simulink model "Cruise_Control"  (R2022b)
settings: configuration reference "CommonModelConfiguration" (kept outside this file)
undefined symbols (not defined in the file): cc_param_23, LCFG_ActivationDeactivation, LCFG_CC_IntStsDelay, LCFG_CC_Tmr1, LCFG_CC_Tmr2, LCFG_DSF_Timeout
settings Model: Creator=RPETE142  LastModifiedBy=OTHOMSO1
settings ConfigSetRef: SourceName=CommonModelConfiguration  SourceLocation=Base Workspace

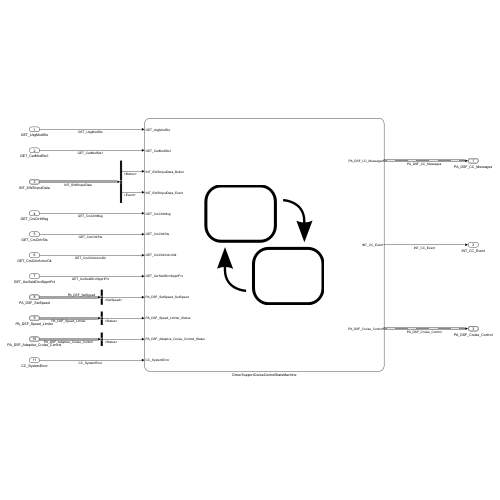
[thumbnail: Simulink's stored preview of the top-level diagram]
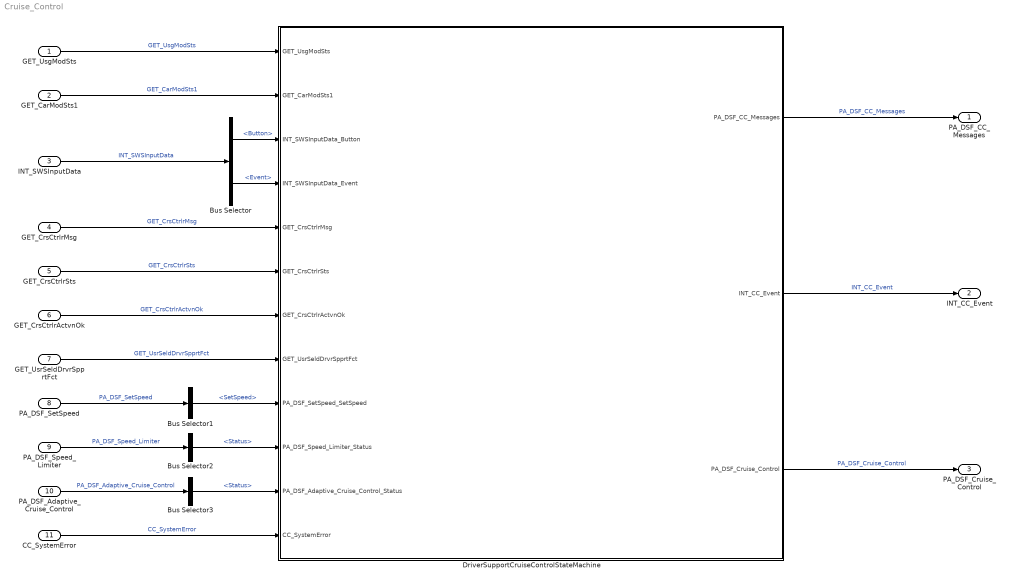
== system Cruise_Control ==
  GET_UsgModSts : Inport  OutDataTypeStr=Enum: UsgModSts1
  GET_CarModSts1 : Inport  Port=2  OutDataTypeStr=Enum: CarModSts1
  INT_SWSInputData : Inport  Port=3  OutDataTypeStr=Bus: SWSInputData  LockScale=on
  GET_CrsCtrlrMsg : Inport  Port=4  OutDataTypeStr=Enum: CrsCtrlrMsg1
  GET_CrsCtrlrSts : Inport  Port=5  OutDataTypeStr=Enum: CrsCtrlrSts1
  GET_CrsCtrlrActvnOk : Inport  Port=6  OutDataTypeStr=Enum: OnOff1
  GET_UsrSeldDrvrSpprtFct : Inport  Port=7  OutDataTypeStr=Enum: DrvrSpprtFct
  PA_DSF_SetSpeed : Inport  Port=8  OutDataTypeStr=Bus: PA_StatusAndValueAndDoubleAndDouble
  PA_DSF_Speed_Limiter : Inport  Port=9  OutDataTypeStr=Bus: PA_DSF
  PA_DSF_Adaptive_Cruise_Control : Inport  Port=10  OutDataTypeStr=Bus: PA_DSF_ACC
  CC_SystemError : Inport  Port=11  OutDataTypeStr=boolean
  Bus Selector : BusSelector  OutputSignals=Button,Event
  Bus Selector1 : BusSelector  OutputSignals=SetSpeed
  Bus Selector2 : BusSelector  OutputSignals=Status
  Bus Selector3 : BusSelector  OutputSignals=Status
  "DriverSupportCruiseControlStateMachine " : Stateflow chart  TreatAsAtomicUnit=on
  PA_DSF_CC_Messages : Outport  OutDataTypeStr=Bus: PA_DSF_Message  VectorParamsAs1DForOutWhenUnconnected=off  LockScale=on
  INT_CC_Event : Outport  Port=2  OutDataTypeStr=Enum: E_DSF_Event  VectorParamsAs1DForOutWhenUnconnected=off
  PA_DSF_Cruise_Control : Outport  Port=3  OutDataTypeStr=Bus: PA_DSF  VectorParamsAs1DForOutWhenUnconnected=off
  wires:
  GET_UsgModSts/1 -> "DriverSupportCruiseControlStateMachine "/1(GET_UsgModSts)  "GET_UsgModSts"
  GET_CarModSts1/1 -> "DriverSupportCruiseControlStateMachine "/2(GET_CarModSts1)  "GET_CarModSts1"
  GET_CrsCtrlrMsg/1 -> "DriverSupportCruiseControlStateMachine "/5(GET_CrsCtrlrMsg)  "GET_CrsCtrlrMsg"
  GET_CrsCtrlrActvnOk/1 -> "DriverSupportCruiseControlStateMachine "/7(GET_CrsCtrlrActvnOk)  "GET_CrsCtrlrActvnOk"
  GET_CrsCtrlrSts/1 -> "DriverSupportCruiseControlStateMachine "/6(GET_CrsCtrlrSts)  "GET_CrsCtrlrSts"
  "DriverSupportCruiseControlStateMachine "/1(PA_DSF_CC_Messages) -> PA_DSF_CC_Messages/1  "PA_DSF_CC_Messages"
  "DriverSupportCruiseControlStateMachine "/2(INT_CC_Event) -> INT_CC_Event/1  "INT_CC_Event"
  "DriverSupportCruiseControlStateMachine "/3(PA_DSF_Cruise_Control) -> PA_DSF_Cruise_Control/1  "PA_DSF_Cruise_Control"
  GET_UsrSeldDrvrSpprtFct/1 -> "DriverSupportCruiseControlStateMachine "/8(GET_UsrSeldDrvrSpprtFct)  "GET_UsrSeldDrvrSpprtFct"
  PA_DSF_SetSpeed/1 -> Bus Selector1/1  "PA_DSF_SetSpeed"
  PA_DSF_Speed_Limiter/1 -> Bus Selector2/1  "PA_DSF_Speed_Limiter"
  PA_DSF_Adaptive_Cruise_Control/1 -> Bus Selector3/1  "PA_DSF_Adaptive_Cruise_Control"
  CC_SystemError/1 -> "DriverSupportCruiseControlStateMachine "/12(CC_SystemError)  "CC_SystemError"
  INT_SWSInputData/1 -> Bus Selector/1  "INT_SWSInputData"
  Bus Selector/2 -> "DriverSupportCruiseControlStateMachine "/4(INT_SWSInputData_Event)  "<Event>"
  Bus Selector/1 -> "DriverSupportCruiseControlStateMachine "/3(INT_SWSInputData_Button)  "<Button>"
  Bus Selector1/1 -> "DriverSupportCruiseControlStateMachine "/9(PA_DSF_SetSpeed_SetSpeed)  "<SetSpeed>"
  Bus Selector2/1 -> "DriverSupportCruiseControlStateMachine "/10(PA_DSF_Speed_Limiter_Status)  "<Status>"
  Bus Selector3/1 -> "DriverSupportCruiseControlStateMachine "/11(PA_DSF_Adaptive_Cruise_Control_Status)  "<Status>"

== stateflow chart Cruise_Control/DriverSupportCruiseControlStateMachine  ==
  state CARCONFIG_INVALID
    entry:
    INT_CC_Event = E_DSF_Event.NoReq;
    PA_DSF_Cruise_Control.Status=E_CommonStatus.NotPresent;
    PA_DSF_Cruise_Control.Value=E_DSF_Value.DSF_Selected;
    PA_DSF_CC_Messages.Status = E_CommonStatus.NotPresent;
    PA_DSF_CC_Messages.Value = E_DSF_Messages.Messages_Off;
  state SYSTEM_OK
    state isActive = activationCheck [function]
      (default) -> (junction 35)
      (junction 35) -> (junction 28) [order 1] : [GET_UsgModSts == UsgModSts1.UsgModSts1_UsgModDrvg && ...
          | (GET_CarModSts1 == CarModSts1.CarModSts1_CarModNorm ||...
          | GET_CarModSts1 == CarModSts1.CarModSts1_CarModDyno) &&...
          | (GET_UsrSeldDrvrSpprtFct==DrvrSpprtFct.DrvrSpprtFct_CC ||...
          | PA_DSF_Cruise_Control.Value==E_DSF_Value.DSF_Active) &&...
          | PA_DSF_Speed_Limiter_Status ~=E_CommonStatus.Available &&...
          | PA_DSF_Adaptive_Cruise_Control_Status~=E_CommonStatus.Available]
      (junction 35) -> (junction 29) [order 2] : {isActive = false;}
      (junction 28) -> (junction 30) : {isActive = true;}
      (junction 30) -> (junction 29)
      (junction 29) -> (junction 31)
    state NOT_ACTIVE
      entry:
      INT_CC_Event = E_DSF_Event.NoReq;
      PA_DSF_Cruise_Control.Status=E_CommonStatus.Disabled;
      PA_DSF_CC_Messages.Status = E_CommonStatus.Disabled;
      state MESSAGES_OFF
        entry:
        PA_DSF_CC_Messages.Value=E_DSF_Messages.Messages_Off;
        PA_DSF_Cruise_Control.Value=E_DSF_Value.DSF_Selected;
      state CANCEL_WARNING
        entry:
        PA_DSF_CC_Messages.Value=E_DSF_Messages.Messages_CancelWarning;
        PA_DSF_Cruise_Control.Value=E_DSF_Value.DSF_Selected;
      (default) -> (junction 1215)
      (junction 1215) -> (junction 1214) [order 1] : [PA_DSF_Cruise_Control.Value==E_DSF_Value.DSF_Active]
      (junction 1215) -> MESSAGES_OFF [order 2]
      (junction 1214) -> SYSTEM_OK.NOT_ACTIVE.CANCEL_WARNING
      SYSTEM_OK.NOT_ACTIVE.CANCEL_WARNING -> MESSAGES_OFF : [after(LCFG_DSF_Timeout, sec)]
    state PENDING
    state PENDING1
    state ACTIVE
      state MESSAGES [parallel]
        entry:
        PA_DSF_CC_Messages.Status = E_CommonStatus.Available;
        settings: executionOrder=1
        state retVal = ccMessages [function]
          state retVal2 = ccActivationReq [function]
            (default) -> (junction 1536)
            (junction 1536) -> (junction 1537) [order 1] : [(GET_CrsCtrlrSts ~= CrsCtrlrSts1.CrsCtrlrSts1_Actv)...
                | && (GET_CrsCtrlrActvnOk == OnOff1.OnOff1_Off)...
                | && (INT_SWSInputData_Button ==  E_SWSButton.BtnL1Req)...
                | && hasChangedTo(INT_SWSInputData_Event,E_SWSEvent.Push)]
            (junction 1536) -> (junction 1539) [order 2]
            (junction 1537) -> (junction 1538)
            (junction 1539) -> (junction 1538) [order 1] : [(GET_CrsCtrlrSts ~= CrsCtrlrSts1.CrsCtrlrSts1_Actv)...
                | && (GET_CrsCtrlrActvnOk == OnOff1.OnOff1_Off)...
                | && (INT_SWSInputData_Button ==  E_SWSButton.BtnL5Req)...
                | && hasChangedTo(INT_SWSInputData_Event,E_SWSEvent.Push)...
                | && (PA_DSF_SetSpeed_SetSpeed~=0)]
            (junction 1538) -> (junction 1540) : {retVal2 = true;}
            (junction 1539) -> (junction 1541) [order 2] : {retVal2 = false;}
            (junction 1540) -> (junction 1541)
            (junction 1541) -> (junction 1542)
          (default) -> (junction 1502)
          (junction 1502) -> (junction 1487) [order 1] : [hasChangedTo(GET_CrsCtrlrMsg, CrsCtrlrMsg1.CrsCtrlrMsg1_CrsCtrlrCncl)]
              | {PA_DSF_CC_Messages.Value = E_DSF_Messages.Messages_CancelWarning;}
          (junction 1502) -> (junction 1504) [order 2]
          (junction 1487) -> (junction 1484)
          (junction 1504) -> (junction 1484) [order 1] : [hasChangedTo(GET_CrsCtrlrMsg, CrsCtrlrMsg1.CrsCtrlrMsg1_CrsCtrlrCnclSpdLoLimExcdd)]
              | {PA_DSF_CC_Messages.Value = E_DSF_Messages.Messages_CancelLowSpeed;}
          (junction 1504) -> (junction 1506) [order 2]
          (junction 1484) -> (junction 1456)
          (junction 1506) -> (junction 1456) [order 1] : [hasChangedTo(GET_CrsCtrlrMsg, CrsCtrlrMsg1.CrsCtrlrMsg1_OvrdTiMaxExcdd)]
              | {PA_DSF_CC_Messages.Value = E_DSF_Messages.Messages_CancelMaxOverride;}
          (junction 1506) -> (junction 1508) [order 2]
          (junction 1456) -> (junction 1494)
          (junction 1508) -> (junction 1510) [order 1] : [ccActivationReq()]
          (junction 1510) -> (junction 1494) [order 1] : [(GET_CrsCtrlrMsg == CrsCtrlrMsg1.CrsCtrlrMsg1_CrsCtrlrInhb)]
              | {PA_DSF_CC_Messages.Value = E_DSF_Messages.Messages_Unavailable;}
          (junction 1508) -> (junction 1517) [order 2]
          (junction 1510) -> (junction 1512) [order 2]
          (junction 1494) -> (junction 1463)
          (junction 1512) -> (junction 1463) [order 1] : [(GET_CrsCtrlrMsg == CrsCtrlrMsg1.CrsCtrlrMsg1_SpdLoLimExcdd)]
              | {PA_DSF_CC_Messages.Value = E_DSF_Messages.Messages_UnavailableLowSpeed;}
          (junction 1512) -> (junction 1515) [order 2]
          (junction 1463) -> (junction 1458)
          (junction 1515) -> (junction 1517) [order 2]
          (junction 1515) -> (junction 1458) [order 1] : [(GET_CrsCtrlrMsg == CrsCtrlrMsg1.CrsCtrlrMsg1_DrvModSeldNotOk)]
              |  {PA_DSF_CC_Messages.Value = E_DSF_Messages.Messages_UnavailableDriveMode;}
          (junction 1517) -> (junction 1533) : {retVal = false;}
          (junction 1458) -> (junction 1529) : {retVal = true;}
          (junction 1529) -> (junction 1533)
          (junction 1533) -> (junction 1531)
        state HIDE_MESSAGES
          entry: PA_DSF_CC_Messages.Value = E_DSF_Messages.Messages_Off;
        state SHOW_MESSAGES
        (default) -> HIDE_MESSAGES
        HIDE_MESSAGES -> SHOW_MESSAGES : [ccMessages()]
        SHOW_MESSAGES -> HIDE_MESSAGES [order 2] : [after(LCFG_DSF_Timeout,sec) ||...
            |  (GET_CrsCtrlrMsg == CrsCtrlrMsg1.CrsCtrlrMsg1_BrkOvrheatd) || ...
            | hasChangedTo(GET_CrsCtrlrSts,CrsCtrlrSts1.CrsCtrlrSts1_Actv)]
        SHOW_MESSAGES -> SHOW_MESSAGES [order 1] : [ccMessages()]
      state CC [parallel]
        entry: PA_DSF_Cruise_Control.Status=E_CommonStatus.Available;
        settings: executionOrder=2
        state STANDBY
          entry:
          PA_DSF_Cruise_Control.Value=E_DSF_Value.DSF_Standby;
          state NO_EVENT
            entry: INT_CC_Event=E_DSF_Event.NoReq;
          state EVENT
          (default) -> SYSTEM_OK.ACTIVE.CC.STANDBY.EVENT
          SYSTEM_OK.ACTIVE.CC.STANDBY.EVENT -> SYSTEM_OK.ACTIVE.CC.STANDBY.NO_EVENT : [after(LCFG_ActivationDeactivation,sec)]
        state SELECTED
          entry:
          PA_DSF_Cruise_Control.Value=E_DSF_Value.DSF_Selected;
        state ON
          entry:
          PA_DSF_Cruise_Control.Value=E_DSF_Value.DSF_Active;
          state NO_EVENT
            entry: INT_CC_Event=E_DSF_Event.NoReq;
          state EVENT
          (default) -> SYSTEM_OK.ACTIVE.CC.ON.EVENT
          SYSTEM_OK.ACTIVE.CC.ON.EVENT -> SYSTEM_OK.ACTIVE.CC.ON.NO_EVENT : [after(LCFG_ActivationDeactivation,sec)]
        (default) -> SELECTED
        SELECTED -> ON [order 2] : [(after(LCFG_CC_IntStsDelay, sec) &&...
            | GET_CrsCtrlrSts==CrsCtrlrSts1.CrsCtrlrSts1_Actv)]
        SELECTED -> ON [order 1] : [INT_SWSInputData_Button==E_SWSButton.BtnL1Req &&...
            | hasChangedTo(INT_SWSInputData_Event,E_SWSEvent.Push) &&...
            | GET_CrsCtrlrActvnOk==OnOff1.OnOff1_On]
            | {INT_CC_Event=E_DSF_Event.Activation;}
        STANDBY -> ON [order 3] : [(after(LCFG_CC_IntStsDelay, sec) &&...
            | GET_CrsCtrlrSts==CrsCtrlrSts1.CrsCtrlrSts1_Actv)]
        STANDBY -> ON [order 1] : [INT_SWSInputData_Button==E_SWSButton.BtnL1Req &&...
            | hasChangedTo(INT_SWSInputData_Event,E_SWSEvent.Push) &&...
            | GET_CrsCtrlrActvnOk==OnOff1.OnOff1_On &&...
            | INT_CC_Event==E_DSF_Event.NoReq]
            | {INT_CC_Event=E_DSF_Event.Activation;}
        STANDBY -> ON [order 2] : [INT_SWSInputData_Button==E_SWSButton.BtnL5Req &&...
            | hasChangedTo(INT_SWSInputData_Event, E_SWSEvent.Push) &&...
            | GET_CrsCtrlrActvnOk==OnOff1.OnOff1_On &&...
            | PA_DSF_SetSpeed_SetSpeed~=0 &&...
            | INT_CC_Event==E_DSF_Event.NoReq]
            | {INT_CC_Event=E_DSF_Event.Resume;}
        ON -> STANDBY [order 1] : [(INT_SWSInputData_Button==E_SWSButton.BtnL1Req &&...
            | hasChangedTo(INT_SWSInputData_Event, E_SWSEvent.Push) &&...
            | INT_CC_Event==E_DSF_Event.NoReq) ||...
            | INT_SWSInputData_Event == E_SWSEvent.Deactivation]
            | {INT_CC_Event=E_DSF_Event.Deactivation;}
        ON -> STANDBY [order 2] : [(after(LCFG_CC_IntStsDelay, sec) &&...
            | GET_CrsCtrlrSts~=CrsCtrlrSts1.CrsCtrlrSts1_Actv)]
    (default) -> NOT_ACTIVE
    NOT_ACTIVE -> PENDING : [activationCheck()]
    PENDING -> NOT_ACTIVE [order 2] : [~activationCheck()]
    PENDING1 -> NOT_ACTIVE [order 1] : [~activationCheck()&&...
        | after(LCFG_CC_Tmr1,sec)]
    PENDING -> ACTIVE [order 1] : [activationCheck()&&...
        | after(LCFG_CC_Tmr2,sec)]
    PENDING1 -> ACTIVE [order 2] : [activationCheck()]
    ACTIVE -> PENDING1 : [~activationCheck()]
  state SYSTEM_ERROR
    entry: PA_DSF_Cruise_Control.Status=E_CommonStatus.SystemError;
    PA_DSF_CC_Messages.Status=E_CommonStatus.SystemError;
    INT_CC_Event=E_DSF_Event.NoReq;
    state retVal = ccActivationReq [function]
      (default) -> (junction 1233)
      (junction 1233) -> (junction 1234) [order 1] : [(INT_SWSInputData_Button==E_SWSButton.BtnL1Req ||...
          | (INT_SWSInputData_Button==E_SWSButton.BtnL5Req && ...
          | PA_DSF_SetSpeed_SetSpeed~=0)) &&...
          | hasChangedTo(INT_SWSInputData_Event, E_SWSEvent.Push) &&...
          | GET_UsrSeldDrvrSpprtFct==DrvrSpprtFct.DrvrSpprtFct_CC]
      (junction 1234) -> (junction 1236) : {retVal=true;}
      (junction 1233) -> (junction 1235) [order 2] : {retVal=false;}
      (junction 1236) -> (junction 1235)
      (junction 1235) -> (junction 1237)
    state CANCEL_WARNING
      entry:
      PA_DSF_CC_Messages.Value=E_DSF_Messages.Messages_CancelWarning;
      PA_DSF_Cruise_Control.Value=E_DSF_Value.DSF_Selected;
    state UNAVAILABLE
      entry:
      PA_DSF_CC_Messages.Value=E_DSF_Messages.Messages_Unavailable;
    state NO_MESSAGES
      entry:
      PA_DSF_CC_Messages.Value=E_DSF_Messages.Messages_Off;
      PA_DSF_Cruise_Control.Value=E_DSF_Value.DSF_Selected;
    (default) -> (junction 1224)
    (junction 1224) -> (junction 1218) [order 1] : [PA_DSF_Cruise_Control.Value==E_DSF_Value.DSF_Active]
    (junction 1224) -> NO_MESSAGES [order 2]
    (junction 1218) -> SYSTEM_ERROR.CANCEL_WARNING
    UNAVAILABLE -> UNAVAILABLE [order 2] : [ccActivationReq()]
    SYSTEM_ERROR.CANCEL_WARNING -> UNAVAILABLE [order 2] : [ccActivationReq()]
    UNAVAILABLE -> NO_MESSAGES [order 1] : [after(LCFG_DSF_Timeout, sec)]
    NO_MESSAGES -> UNAVAILABLE : [ccActivationReq()]
    SYSTEM_ERROR.CANCEL_WARNING -> NO_MESSAGES [order 1] : [after(LCFG_DSF_Timeout, sec)]
  (default) -> (junction 284)
  (junction 284) -> CARCONFIG_INVALID [order 2]
  (junction 284) -> (junction 287) [order 1] : [cc_param_23 > 1]
      | {PA_DSF_Cruise_Control.Value=E_DSF_Value.DSF_Selected;}
  (junction 287) -> SYSTEM_OK [order 2]
  (junction 287) -> (junction 1168) [order 1] : [CC_SystemError == true ||...
      |  INT_SWSInputData_Event == E_SWSEvent.ButtonStuck]
  SYSTEM_OK -> SYSTEM_ERROR : [CC_SystemError == true ||...
      |  INT_SWSInputData_Event == E_SWSEvent.ButtonStuck]
  SYSTEM_ERROR -> SYSTEM_OK : [CC_SystemError == false &&...
      |  INT_SWSInputData_Event ~= E_SWSEvent.ButtonStuck]
  (junction 1168) -> SYSTEM_ERROR
  data: isActive function_output; retVal2 function_output; retVal function_output; retVal function_output; cc_param_23 parameter double; GET_UsgModSts input Enum: UsgModSts1; GET_CarModSts1 input Enum: CarModSts1; INT_SWSInputData_Button input Enum: E_SWSButton; INT_SWSInputData_Event input Enum: E_SWSEvent; PA_DSF_CC_Messages output Bus: PA_DSF_Message =0; LCFG_CC_Tmr1 parameter double; LCFG_DSF_Timeout parameter double; LCFG_CC_Tmr2 parameter double; LCFG_CC_IntStsDelay parameter double; INT_CC_Event output Enum: E_DSF_Event; GET_CrsCtrlrMsg input Enum: CrsCtrlrMsg1; PA_DSF_Cruise_Control output Bus: PA_DSF =0; GET_CrsCtrlrSts input Enum: CrsCtrlrSts1; GET_CrsCtrlrActvnOk input Enum: OnOff1; GET_UsrSeldDrvrSpprtFct input Enum: DrvrSpprtFct; PA_DSF_SetSpeed_SetSpeed input double; PA_DSF_Speed_Limiter_Status input Enum: E_CommonStatus; PA_DSF_Adaptive_Cruise_Control_Status input Enum: E_CommonStatus; CC_SystemError input boolean; LCFG_ActivationDeactivation parameter double
